simulink model "model_induction_Motor_V_F_Control_v1"  (R2017b)
settings: Solver=ode45  StartTime=0.0  StopTime=10  MaxStep=1e-4  RelTol=1e-3
libraries: powerlib x6, simulink x1
settings Model: SimulationMode=accelerator  Creator=proso  LastModifiedBy=proso

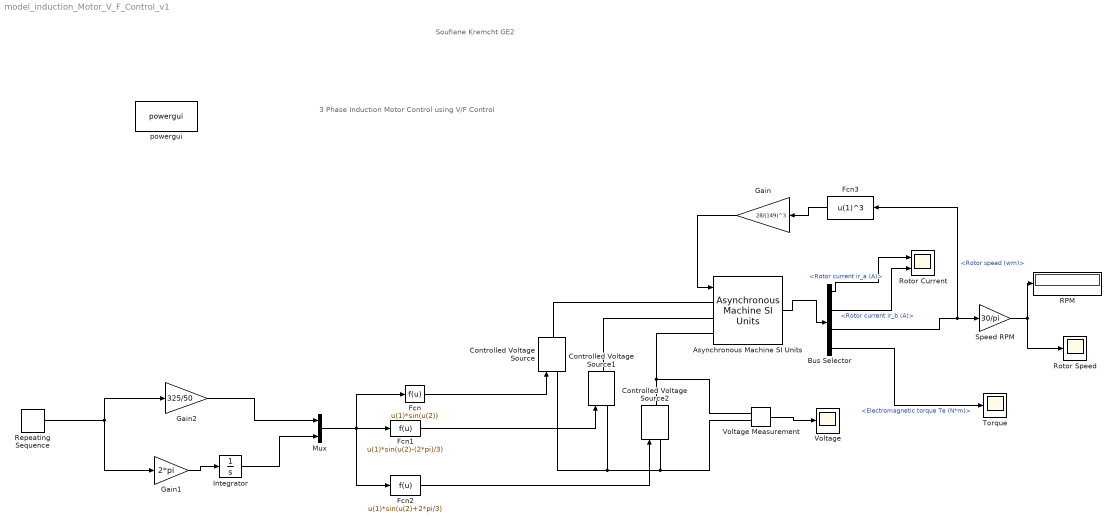
== system model_induction_Motor_V_F_Control_v1 ==
  note: Soufiane Kremcht GE2
  note: 3 Phase Induction Motor Control using V/F Control
  Asynchronous Machine SI Units : powerlib/Machines/Asynchronous Machine SI Units  RotorType=Squirrel-cage  PresetModel="15:  5.4 HP (4KW)   400 V  50Hz 1430 RPM"  MechanicalLoad=Torque Tm  ShowDetailedParameters=on  ReferenceFrame=Rotor  Units=SI  MeasurementBus=off  NominalParameters=[4000 400 50]  Stator=[1.405 0.005839]  Rotor=[1.395 0.005839]  Cage1=[1.543 0.006067]  Cage2=[3.309 0.005654]  Lm=0.1722  Mechanical=[0.0131 0.002985 2]  PolePairs=2  InitialConditions=[1 0 0 0 0 0 0 0]  SimulateSaturation=off  Saturation=[14.03593122, 27.81365428, 53.79336849, 72.68890987, 97.98006896, 148.6815601, 215.7428561, 302.9841135, 428.7778367 ; 230, 322, 414, 460, 506, 552, 598, 644, 690]  LoadFlowParameters=1492000  TsPowergui=0  TsBlock=-1  IterativeModel=Trapezoidal non iterative  IterativeDiscreteModel=Trapezoidal non iterative  Pmec=1.492e+006
  Bus Selector : BusSelector  OutputSignals=Rotor measurements.Rotor current ir_a (A),Rotor measurements.Rotor current ir_b (A),Mechanical.Rotor speed (wm),Mechanical.Electromagnetic torque Te (N*m)
  Controlled Voltage Source : powerlib/Electrical Sources/Controlled Voltage Source  Initialize=on  Source_Type=AC  Amplitude=0  Phase=0  Frequency=0  Measurements=None
  Controlled Voltage Source1 : powerlib/Electrical Sources/Controlled Voltage Source  Initialize=on  Source_Type=AC  Amplitude=0  Phase=0  Frequency=0  Measurements=None
  Controlled Voltage Source2 : powerlib/Electrical Sources/Controlled Voltage Source  Initialize=on  Source_Type=AC  Amplitude=0  Phase=0  Frequency=0  Measurements=None
  Fcn : Fcn  Expr=u(1)*sin(u(2))
  Fcn1 : Fcn  Expr=u(1)*sin(u(2)-(2*pi)/3)
  Fcn2 : Fcn  Expr=u(1)*sin(u(2)+2*pi/3)
  Fcn3 : Fcn  Expr=u(1)^3
  Gain : Gain  Gain=28/(149)^3
  Gain1 : Gain  Gain=2*pi
  Gain2 : Gain  Gain=325/50
  Integrator : Integrator
  Mux : Mux  Inputs=2
  RPM : Display
  Repeating Sequence : simulink/Sources/Repeating Sequence  rep_seq_t=[0 .1 10]  rep_seq_y=[0 50 50]
  Rotor Current : Scope  NumInputPorts=2
  Rotor Speed : Scope
  Speed RPM : Gain  Gain=30/pi
  "Torque " : Scope
  Voltage : Scope
  Voltage Measurement : powerlib/Measurements/Voltage Measurement  PhasorSimulation=off  OutputType=Complex  PSBequivalent=0
  powergui : powerlib/powergui  Priority=1  SimulationMode=Continuous  SampleTime=10e-5  frequency=60  Iterations=50  frequencyindice=0  Pbase=100e6  ErrMax=1e-4  UnitsV=kV  UnitsW=MW  buscounter=0  FunctionMessages=off  echomessages=off  EnableUseOfTLC=off  CurrentSourceSwitches=off  DisableSnubberDevices=off  DisableRonSwitches=off  DisableVfSwitches=off  DisplayEquations=off  SolverType=Tustin/Backward Euler (TBE)  Interpol=off  ExternalGateDelay=off  methode=off  Ts=100  x0status=blocks  SPID=on  SwTol=0  HookPort=off  RestoreLinks=warning  ResistiveCurrentMeasurement=off  Frange=[0:2:500]  Ylog=off  Xlog=on  ShowGrid=off  save=off  variable=ZData  structure=0  ZoomFFT=off  StartTime=0.0  cycles=1  DisplayStyle=1  fundamental=60  FreqAxis=off  MaxFrequency=1000  frequencyindicesteady=1  RmsSteady=1  display=off
  wires:
  Asynchronous Machine SI Units/1 -> Bus Selector/1
  Bus Selector/1 -> Rotor Current/1  "<Rotor current ir_a (A)>"
  Bus Selector/2 -> Rotor Current/2  "<Rotor current ir_b (A)>"
  Bus Selector/4 -> "Torque "/1  "<Electromagnetic torque Te (N*m)>"
  Speed RPM/1 -> RPM/1, Rotor Speed/1
  Bus Selector/3 -> Fcn3/1, Speed RPM/1  "<Rotor speed (wm)>"
  Gain/1 -> Asynchronous Machine SI Units/1
  Fcn/1 -> Controlled Voltage Source/1
  Fcn1/1 -> Controlled Voltage Source1/1
  Fcn2/1 -> Controlled Voltage Source2/1
  Mux/1 -> Fcn2/1, Fcn1/1, Fcn/1
  Repeating Sequence/1 -> Gain1/1, Gain2/1
  Gain1/1 -> Integrator/1
  Integrator/1 -> Mux/2
  Gain2/1 -> Mux/1
  Voltage Measurement/1 -> Voltage/1
  Fcn3/1 -> Gain/1
  connections:
  Asynchronous Machine SI Units/LConn1 -- Controlled Voltage Source/RConn1
  Asynchronous Machine SI Units/LConn2 -- Controlled Voltage Source1/RConn1
  Asynchronous Machine SI Units/LConn3 -- Voltage Measurement/LConn1 -- Controlled Voltage Source2/RConn1
  Controlled Voltage Source1/LConn1 -- Controlled Voltage Source/LConn1 -- Controlled Voltage Source2/LConn1 -- Voltage Measurement/LConn2
